simulink model "VehicleBackKin"  (R2024b)
settings: Solver=FixedStepAuto  StartTime=0.0  StopTime=inf  FixedStep=VehicleEnv.Ts  RelTol=1e-3
values from neighbouring files (symbols this model uses):
  em = ElectricMotor    [VehicleBackKinEnv.m]
  ess = VehicleEnv.ess    [VehicleBackKinEnv.m]
  fd = FinalDrive    [VehicleBackKinEnv.m]
  gb = Gearbox    [VehicleBackKinEnv.m]
  ice = Engine    [VehicleBackKinEnv.m]
  reward = VehicleEnv.reward    [VehicleBackKinEnv.m]
  selector_in = zeros(size(obs_info.Name))    [VehicleBackKinEnv.m]
  veh = Vehicle    [VehicleBackKinEnv.m]
  VehicleEnv = evalin("base","VehicleEnv")    [VehicleBackKinEnv.m]
  wh = Wheels    [VehicleBackKinEnv.m]
undefined symbols (not defined in the file or in its folder): agentSampleTime, cycle_insimulink, cycleTime, transfer_fun_coeff
libraries: simulink x3, rllib x1, autolibsharedcoreengin x1
(part 4 of 4)

== system VehicleBackKin/Vehicle environment/Vehicle dynamics/Final drive power computation-ICE on/Vehicle equivalent mass ==
  note: Wheel
  note: ICE
  note: EM
  In2 : Inport
  data2 : Inport  Port=2
  Add : Sum
  Add1 : Sum  Inputs=++++
  Constant : Constant  Value=0
  Constant2 : Constant  Value=veh.mass
  Constant3 : Constant  Value=wh.inertiaR
  Constant4 : Constant  Value=wh.inertiaF
  Constant5 : Constant  Value=wh.radius
  Constant6 : Constant  Value=ice.inertia
  Constant7 : Constant  Value=fd.ratio
  Constant8 : Constant  Value=em.inertia
  Constant9 : Constant  Value=em.gear_ratio
  Divide : Product  Inputs=*/
  Divide1 : Product  Inputs=/*
  Divide2 : Product  Inputs=/*
  Gain : Gain  Gain=2
  Product : Product
  Product1 : Product
  Product2 : Product  Inputs=3
  Square : Math  Operator=square
  Square1 : Math  Operator=square
  Square2 : Math  Operator=square
  Switch : Switch  Criteria=u2 > Threshold  SaturateOnIntegerOverflow=off  InputSameDT=off
  Out1 : Outport
  wires:
  Constant3/1 -> Add/1
  Square1/1 -> Product2/1, Product1/2
  Divide/1 -> Add1/2
  Constant4/1 -> Add/2
  Product2/1 -> Divide2/2
  Constant5/1 -> Square/1
  Product/1 -> Square1/1
  Constant8/1 -> Product2/2
  Switch/1 -> Add1/3
  Constant/1 -> Switch/3
  Add/1 -> Gain/1
  Divide1/1 -> Switch/1
  Divide2/1 -> Add1/4
  Gain/1 -> Divide/1
  Square/1 -> Divide2/1, Divide1/1, Divide/2
  Square2/1 -> Product2/3
  Constant9/1 -> Square2/1
  Product1/1 -> Divide1/2
  In2/1 -> Product/2  "gear_ratio"
  Add1/1 -> Out1/1  "veh_eq_mass"
  data2/1 -> Switch/2  "ice_state"
  Constant2/1 -> Add1/1
  Constant6/1 -> Product1/1
  Constant7/1 -> Product/1

== matlab function VehicleBackKin/Reinforcement Learning controller/States normalization ==
  data: states input; obs output; states_max parameter; lower parameter; upper parameter; states_min parameter
function obs = fcn(states,states_max,lower,upper,states_min)

obs = (states-states_min)./(states_max-states_min)*(upper-lower)+lower;

== stateflow chart VehicleBackKin/Vehicle environment/ECU/Powertrain power supervisory controller ==
  state Idle
    ice_pwr_dmd = 0;
    em_pwr_dmd = 0;
    state = 0;
  state Traction
    ice_pwr_dmd = ice_pwr_trac;
    em_pwr_dmd = em_pwr_trac;
    state = 1;
  state Braking
    ice_pwr_dmd = 0;
    em_pwr_dmd = em_pwr_reg;
    state = 2;
  (default) -> Idle
  Idle -> Traction : [veh_spd>=0.1]
  Traction -> Idle [order 2] : [veh_spd<0.1]
  Braking -> Idle [order 1] : [veh_spd<0.1]
  Traction -> Braking [order 1] : [pwr_dmd<=0]
  Braking -> Traction [order 2] : [pwr_dmd>0]
  data: ice_pwr_dmd output; ice_pwr_trac input; em_pwr_trac input; pwr_dmd input; veh_spd input; em_pwr_reg input; em_pwr_dmd output; state local
